simulink model "lab2_3"  (Simulink 7.9)
settings: Solver=ode45  StartTime=0.0  StopTime=0.3  RelTol=1e-3
libraries: simulink x2
settings Model: Creator=Aquirel  LastModifiedBy=Aquirel

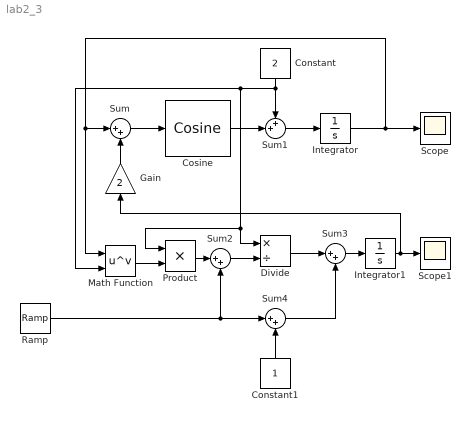
== system lab2_3 ==
  Constant : Constant  Value=2
  Constant1 : Constant
  Cosine : simulink/Lookup Tables/Cosine  Formula=cos(2*pi*u)  NumDataPoints=(2^5)+1  OutputWordLength=16
  Divide : Product  Inputs=*/
  Gain : Gain  Gain=2
  Integrator : Integrator  InitialCondition=1
  Integrator1 : Integrator  InitialCondition=0.05
  Math Function : Math  Operator=pow  SaturateOnIntegerOverflow=on
  Product : Product  RndMeth=Zero
  Ramp : simulink/Sources/Ramp  slope=1  start=0  X0=0
  Scope : Scope
      settings: YMin=0  YMax=2
  Scope1 : Scope
      settings: YMin=0  YMax=2
  Sum{,2..4} (4 alike) : Sum  Inputs=|++
  Sum1 : Sum  Inputs=++|
  wires:
  Sum/1 -> Cosine/1
  Cosine/1 -> Sum1/2
  Constant/1 -> Sum1/1, Math Function/2, Divide/1, Product/1
  Sum1/1 -> Integrator/1
  Integrator/1 -> Scope/1, Sum/1, Math Function/1
  Sum2/1 -> Divide/2
  Math Function/1 -> Product/2
  Product/1 -> Sum2/1
  Ramp/1 -> Sum2/2, Sum4/1
  Divide/1 -> Sum3/1
  Sum4/1 -> Sum3/2
  Constant1/1 -> Sum4/2
  Sum3/1 -> Integrator1/1
  Integrator1/1 -> Scope1/1, Gain/1
  Gain/1 -> Sum/2
